simulink model "rbarm_plan_control_backup"  (R2021a)
settings: Solver=VariableStepAuto  StartTime=0.0  StopTime=6  FixedStep=0.00001  RelTol=1e-3
model workspace: external: MATLAB File E:\attachments\attachments\Assem1_DataFile1.m (data not in the file)
undefined symbols (not defined in the file): smiData, X, Y, Z
libraries: sm_lib x20, nesl_utility x8, simulink x1
settings Model: Creator=Admin  LastModifiedBy=Admin

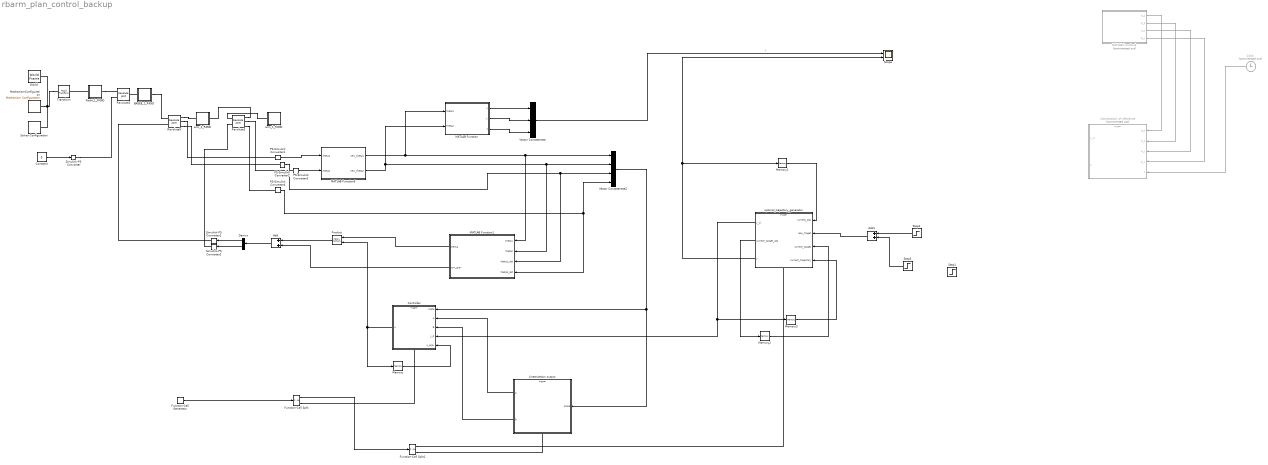
== system rbarm_plan_control_backup ==
  Add : Sum
  Add1 : Sum
  BASEE_1_RIGID : Subsystem
  Clock : Clock  Commented=on
  Constant : Constant  Value=0
  Controller : Subsystem  TreatAsAtomicUnit=on
  Demux : Demux  Outputs=2
  Function-Call Generator : simulink/Ports & Subsystems/Function-Call Generator  sample_time=0.01  numberOfIterations=1  DisallowWideOutput=off
  Function-Call Split : FunctionCallSplit  IconShape=distinctive  NumOutputPorts=2  OutputPortLayout=default
  Function-Call Split1 : FunctionCallSplit  IconShape=distinctive  NumOutputPorts=2  OutputPortLayout=default
  Linearization output : Subsystem  TreatAsAtomicUnit=on
  MATLAB Function : MATLAB Function  TreatAsAtomicUnit=on
  MATLAB Function1 : MATLAB Function  TreatAsAtomicUnit=on
  MATLAB Function3 : MATLAB Function  Commented=on  TreatAsAtomicUnit=on
  MATLAB Function6 : MATLAB Function  TreatAsAtomicUnit=on
  MechanismConfiguration : sm_lib/Utilities/Mechanism Configuration  UniformGravity=Constant  GravityVector=[0 0 9.80665]  GravityVectorUnits=m/s^2  GravityUnits=m/s^2  LinearizationDelta=0.001  JointModeTransitionNonlinearIterations=2
  Memory : Memory  InitialCondition=[0;0]
  Memory1 : Memory  InitialCondition=[0;0;0.24]
  Memory2 : Memory  InitialCondition=[0;0;0.24]
  Memory3 : Memory  InitialCondition=zeros(600,1)
  PS-Simulink Converter{1..4} (4 alike) : nesl_utility/PS-Simulink Converter  PhysicalDomain=network_engine_domain  SubClassName=ps_output  LeftPortType=input  RightPortType=output  PseudoPeriodic=off  Frequencies=[]  Unit=inherit  AffineConversion=off
      settings: SourceProductBaseCode=PW,SS
  Part4_1_RIGID : Subsystem
  Product : Product  Multiplication=Matrix(*)
  Revolute2 : sm_lib/Joints/Revolute Joint  JointMode=Normal  SenseConstraintForce=off  SenseConstraintForceX=off  SenseConstraintForceY=off  SenseConstraintForceZ=off  SenseConstraintTorque=off  SenseConstraintTorqueX=off  SenseConstraintTorqueY=off  SenseConstraintTorqueZ=off  SenseTotalForce=off  SenseTotalForceX=off  SenseTotalForceY=off  SenseTotalForceZ=off  SenseTotalTorque=off  SenseTotalTorqueX=off  SenseTotalTorqueY=off  SenseTotalTorqueZ=off  CompositeWrenchDir=FollowerOnBase  CompositeWrenchFrame=BaseFrame  EquilibriumPosition=0  EquilibriumPositionUnits=deg  SpringStiffness=0  SpringStiffnessUnits=N*m/deg  DampingCoefficient=100  DampingCoefficientUnits=N*m/(deg/s)  TorqueActuationMode=ComputedTorque  MotionActuationMode=InputMotion  SensePosition=off  SenseVelocity=off  SenseAcceleration=off  SenseTorqueForce=off  SenseLowerLimitTorqueForce=off  SenseUpperLimitTorqueForce=off  LowerLimitSpecify=off  LowerLimitBound=-90  LowerLimitBoundUnits=deg  LowerLimitStiffness=1e4  LowerLimitStiffnessUnits=N*m/deg  LowerLimitDamping=10  LowerLimitDampingUnits=N*m/(deg/s)  LowerLimitTransitionRegionWidth=0.1  LowerLimitTransitionRegionWidthUnits=deg  UpperLimitSpecify=off  UpperLimitBound=90  UpperLimitBoundUnits=deg  UpperLimitStiffness=1e4  UpperLimitStiffnessUnits=N*m/deg  UpperLimitDamping=10  UpperLimitDampingUnits=N*m/(deg/s)  UpperLimitTransitionRegionWidth=0.1  UpperLimitTransitionRegionWidthUnits=deg  PositionTargetSpecify=off  PositionTargetPriority=Low  PositionTargetValue=smiData.RevoluteJoint(3).Rz.Pos  PositionTargetValueUnits=deg  VelocityTargetSpecify=off  VelocityTargetPriority=High  VelocityTargetValue=0  VelocityTargetValueUnits=deg/s
  Revolute3 : sm_lib/Joints/Revolute Joint  JointMode=Normal  SenseConstraintForce=off  SenseConstraintForceX=off  SenseConstraintForceY=off  SenseConstraintForceZ=off  SenseConstraintTorque=off  SenseConstraintTorqueX=off  SenseConstraintTorqueY=off  SenseConstraintTorqueZ=off  SenseTotalForce=off  SenseTotalForceX=off  SenseTotalForceY=off  SenseTotalForceZ=off  SenseTotalTorque=off  SenseTotalTorqueX=off  SenseTotalTorqueY=off  SenseTotalTorqueZ=off  CompositeWrenchDir=FollowerOnBase  CompositeWrenchFrame=BaseFrame  EquilibriumPosition=0  EquilibriumPositionUnits=deg  SpringStiffness=0  SpringStiffnessUnits=N*m/deg  DampingCoefficient=0  DampingCoefficientUnits=N*m/(deg/s)  TorqueActuationMode=InputTorque  MotionActuationMode=ComputedMotion  SensePosition=on  SenseVelocity=on  SenseAcceleration=off  SenseTorqueForce=off  SenseLowerLimitTorqueForce=off  SenseUpperLimitTorqueForce=off  LowerLimitSpecify=off  LowerLimitBound=-90  LowerLimitBoundUnits=deg  LowerLimitStiffness=1e4  LowerLimitStiffnessUnits=N*m/deg  LowerLimitDamping=10  LowerLimitDampingUnits=N*m/(deg/s)  LowerLimitTransitionRegionWidth=0.1  LowerLimitTransitionRegionWidthUnits=deg  UpperLimitSpecify=off  UpperLimitBound=90  UpperLimitBoundUnits=deg  UpperLimitStiffness=1e4  UpperLimitStiffnessUnits=N*m/deg  UpperLimitDamping=10  UpperLimitDampingUnits=N*m/(deg/s)  UpperLimitTransitionRegionWidth=0.1  UpperLimitTransitionRegionWidthUnits=deg  PositionTargetSpecify=off  PositionTargetPriority=Low  PositionTargetValue=smiData.RevoluteJoint(4).Rz.Pos  PositionTargetValueUnits=deg  VelocityTargetSpecify=off  VelocityTargetPriority=High  VelocityTargetValue=0  VelocityTargetValueUnits=deg/s
  Revolute5 : sm_lib/Joints/Revolute Joint  JointMode=Normal  SenseConstraintForce=off  SenseConstraintForceX=off  SenseConstraintForceY=off  SenseConstraintForceZ=off  SenseConstraintTorque=off  SenseConstraintTorqueX=off  SenseConstraintTorqueY=off  SenseConstraintTorqueZ=off  SenseTotalForce=off  SenseTotalForceX=off  SenseTotalForceY=off  SenseTotalForceZ=off  SenseTotalTorque=off  SenseTotalTorqueX=off  SenseTotalTorqueY=off  SenseTotalTorqueZ=off  CompositeWrenchDir=FollowerOnBase  CompositeWrenchFrame=BaseFrame  EquilibriumPosition=0  EquilibriumPositionUnits=deg  SpringStiffness=0  SpringStiffnessUnits=N*m/deg  DampingCoefficient=0  DampingCoefficientUnits=N*m/(deg/s)  TorqueActuationMode=InputTorque  MotionActuationMode=ComputedMotion  SensePosition=on  SenseVelocity=on  SenseAcceleration=off  SenseTorqueForce=off  SenseLowerLimitTorqueForce=off  SenseUpperLimitTorqueForce=off  LowerLimitSpecify=off  LowerLimitBound=-90  LowerLimitBoundUnits=deg  LowerLimitStiffness=1e4  LowerLimitStiffnessUnits=N*m/deg  LowerLimitDamping=10  LowerLimitDampingUnits=N*m/(deg/s)  LowerLimitTransitionRegionWidth=0.1  LowerLimitTransitionRegionWidthUnits=deg  UpperLimitSpecify=off  UpperLimitBound=90  UpperLimitBoundUnits=deg  UpperLimitStiffness=1e4  UpperLimitStiffnessUnits=N*m/deg  UpperLimitDamping=10  UpperLimitDampingUnits=N*m/(deg/s)  UpperLimitTransitionRegionWidth=0.1  UpperLimitTransitionRegionWidthUnits=deg  PositionTargetSpecify=off  PositionTargetPriority=Low  PositionTargetValue=smiData.RevoluteJoint(6).Rz.Pos  PositionTargetValueUnits=deg  VelocityTargetSpecify=off  VelocityTargetPriority=High  VelocityTargetValue=0  VelocityTargetValueUnits=deg/s
  Scope : Scope  NumInputPorts=2
  Simulink-PS Converter : nesl_utility/Simulink-PS Converter  PhysicalDomain=network_engine_domain  SubClassName=ps_input  LeftPortType=input  RightPortType=output  PseudoPeriodic=off  Frequencies=[]  NoiseDistribution=none  NoiseParameters=[]  Unit=1  AffineConversion=off  FilteringAndDerivatives=provide  SimscapeFilterOrder=1  InputFilterTimeConstant=0.001  UdotUserProvided=0
      settings: SourceProductBaseCode=PW,SS
  Simulink-PS Converter1 : nesl_utility/Simulink-PS Converter  PhysicalDomain=network_engine_domain  SubClassName=ps_input  LeftPortType=input  RightPortType=output  PseudoPeriodic=off  Frequencies=[]  NoiseDistribution=none  NoiseParameters=[]  Unit=1  AffineConversion=off  FilteringAndDerivatives=provide  SimscapeFilterOrder=1  InputFilterTimeConstant=0.001  UdotUserProvided=0
      settings: SourceProductBaseCode=PW,SS
  Simulink-PS Converter2 : nesl_utility/Simulink-PS Converter  PhysicalDomain=network_engine_domain  SubClassName=ps_input  LeftPortType=input  RightPortType=output  PseudoPeriodic=off  Frequencies=[]  NoiseDistribution=none  NoiseParameters=[]  Unit=1  AffineConversion=off  FilteringAndDerivatives=provide  SimscapeFilterOrder=1  InputFilterTimeConstant=0.001  UdotUserProvided=0
      settings: SourceProductBaseCode=PW,SS
  Solver Configuration : nesl_utility/Solver Configuration  PhysicalDomain=network_engine_domain  SubClassName=solver  LeftPortType=input  RightPortType=generic  Tones=[]  Harmonics=[]  SimulateNoise=off  Profile=off  UseLocalSampling=off  EnableSwitchedLinearOptims=on  FrequencyDomain=off  UseCCode=off  RelTol=0.001  AbsTol=1e-06  MinStep=1e-09  ToWorkspace=off  RevertToSquareIcSolve=off  NumHomotopyIterations=100  PhasorMode=off  PhasorModeNumHarmonics=1  DoDC=off  ResidualTolerance=1e-09  UseLocalSolver=off  LocalSolverChoice=NE_BACKWARD_EULER_ADVANCER  LocalSolverSampleTime=0.001  DoFixedCost=off  MaxNonlinIter=3  MaxModeIter=2  ComputeImpulses=off  ImpulseIterations=2  LinearAlgebra=auto  EquationFormulation=NE_TIME_EF  DelaysMemoryBudget=1024  AutomaticFiltering=on  FilteringTimeConstant=0.001  PartitionStorageMethod=AS_NEEDED  PartitionMemoryBudget=1024  PartitionMethod=ROBUST
      settings: SourceProductBaseCode=PW,SS
  Step1 : Step  Time=3  Before=[0;0;0]  After=[0;0.0439;-0.0557]  SampleTime=0
  Step2 : Step  Time=0.5  Before=[0;0;0.24]  After=[0;-0.1639;0.1]  SampleTime=0
  Step3 : Step  Time=3  Before=[0;0;0]  After=[0;0.0439;-0.2]  SampleTime=0
  Transform : sm_lib/Frames and Transforms/Rigid Transform  TranslationMethod=Cartesian  TranslationStandardOffset=0  TranslationLengthUnit=mm  TranslationStandardAxis=+Z  TranslationCartesianOffset=smiData.RigidTransform(19).translation  TranslationROffset=0  TranslationROffsetUnits=m  TranslationZOffset=0  TranslationZOffsetUnits=m  TranslationThetaOffset=0  TranslationThetaOffsetUnits=deg  RotationMethod=StandardAxis  RotationAngleUnits=rad  RotationStandardAxis=+Z  RotationAngle=smiData.RigidTransform(19).angle  RotationArbitraryAxis=smiData.RigidTransform(19).axis  FollAlignAxisA=+X  BaseAlignAxisA=+Y  FollAlignAxisB=+Y  BaseAlignAxisB=+Z  RotationSequenceAxes=FollowerAxes  RotationSequence=XYX  RotationSequenceAngles=[0 0 0]  RotationSequenceAnglesUnits=deg  RotationMatrix=[1 0 0; 0 1 0; 0 0 1]
  Vector Concatenate : Concatenate  NumInputs=3
  Vector Concatenate2 : Concatenate  NumInputs=4
  World : sm_lib/Frames and Transforms/World Frame
  arm_1_RIGID : Subsystem
  arm_2_RIGID : Subsystem
  discretization of reference : Subsystem  Commented=on  TreatAsAtomicUnit=on
  optimal_trajectory_generator : Subsystem  TreatAsAtomicUnit=on
  wires:
  Constant/1 -> Simulink-PS Converter/1
  MATLAB Function1/2(cori_grav) -> Add/2
  Add/1 -> Demux/1
  Demux/1 -> Simulink-PS Converter1/1
  Demux/2 -> Simulink-PS Converter2/1
  MATLAB Function/2(y) -> Vector Concatenate/2
  MATLAB Function/1(x) -> Vector Concatenate/1
  MATLAB Function/3(z) -> Vector Concatenate/3
  MATLAB Function1/1(inertia) -> Product/1
  MATLAB Function3/1(a_z) -> discretization of reference/1(a_z)
  MATLAB Function3/2(b_z) -> discretization of reference/2(b_z)
  MATLAB Function3/3(a_y) -> discretization of reference/3(a_y)
  MATLAB Function3/4(b_y) -> discretization of reference/4(b_y)
  Clock/1 -> discretization of reference/5(t)
  Product/1 -> Add/1
  PS-Simulink Converter3/1 -> MATLAB Function6/2(theta2)
  PS-Simulink Converter1/1 -> MATLAB Function6/1(theta1)
  MATLAB Function6/1(new_theta1) -> MATLAB Function1/1(theta1), Vector Concatenate2/1, MATLAB Function/1(theta1)
  MATLAB Function6/2(new_theta2) -> MATLAB Function/2(theta2), MATLAB Function1/2(theta2), Vector Concatenate2/2
  Controller/1(u) -> Product/2, Memory/1
  Function-Call Generator/1 -> Function-Call Split/1
  Function-Call Split/2 -> Controller/Trigger
  Linearization output/1(A) -> Controller/2(A)
  Linearization output/2(B) -> Controller/3(B)
  Vector Concatenate2/1 -> Linearization output/1(state), Controller/1(state)
  Function-Call Split/1 -> Function-Call Split1/1
  PS-Simulink Converter2/1 -> MATLAB Function1/3(theta1_dot), Vector Concatenate2/3
  PS-Simulink Converter4/1 -> MATLAB Function1/4(theta2_dot), Vector Concatenate2/4
  Vector Concatenate/1 -> Scope/1  "Y"
  Memory/1 -> Controller/5(u_prev)
  Step2/1 -> Add1/1
  Add1/1 -> optimal_trajectory_generator/2(new_traget)
  optimal_trajectory_generator/2(current_target_pos) -> Memory2/1
  Memory2/1 -> optimal_trajectory_generator/3(current_target)
  Memory3/1 -> optimal_trajectory_generator/4(current_trajectory)
  optimal_trajectory_generator/3(y) -> Scope/2, Memory1/1
  Function-Call Split1/1 -> optimal_trajectory_generator/Trigger
  Function-Call Split1/2 -> Linearization output/Trigger
  optimal_trajectory_generator/1(y_d) -> Controller/4(y_d), Memory3/1
  Memory1/1 -> optimal_trajectory_generator/1(current_pos)
  Step3/1 -> Add1/2
  connections:
  Transform/LConn1 -- MechanismConfiguration/RConn1 -- Solver Configuration/RConn1 -- World/RConn1
  BASEE_1_RIGID/RConn1 -- Revolute5/LConn1
  Revolute5/RConn1 -- arm_2_RIGID/LConn1
  Part4_1_RIGID/LConn1 -- Transform/RConn1
  Part4_1_RIGID/RConn1 -- Revolute2/LConn1
  BASEE_1_RIGID/LConn1 -- Revolute2/RConn1
  Revolute3/LConn1 -- arm_1_RIGID/LConn1
  Revolute3/RConn1 -- arm_2_RIGID/RConn1
  Simulink-PS Converter/RConn1 -- Revolute2/LConn2
  Revolute5/RConn2 -- PS-Simulink Converter1/LConn1
  Revolute5/RConn3 -- PS-Simulink Converter2/LConn1
  Revolute3/RConn2 -- PS-Simulink Converter3/LConn1
  Revolute3/RConn3 -- PS-Simulink Converter4/LConn1
  Simulink-PS Converter1/RConn1 -- Revolute5/LConn2
  Simulink-PS Converter2/RConn1 -- Revolute3/LConn2

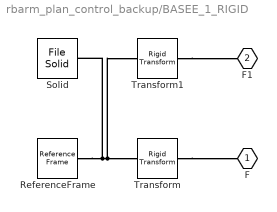
== system rbarm_plan_control_backup/BASEE_1_RIGID ==
  ReferenceFrame : sm_lib/Frames and Transforms/Reference Frame
  Solid : sm_lib/Body Elements/File Solid  ExtGeomFileName=BASEE_Default_sldprt.STEP  UnitType=FromFile  ExtGeomFileUnits=m  StepReaderType=HEX  ExportConvexHullGeometry=off  InertiaType=CalculateFromGeometry  Mass=smiData.Solid(7).mass  MassUnits=kg  CenterOfMass=smiData.Solid(7).CoM  CenterOfMassUnits=mm  MomentsOfInertia=smiData.Solid(7).MoI  MomentsOfInertiaUnits=kg*mm^2  ProductsOfInertia=smiData.Solid(7).PoI  ProductsOfInertiaUnits=kg*mm^2  BasedOnType=Density  Density=8000  DensityUnits=kg/m^3  DoExposeReferenceFrame=on  SerializedFrames=<Frames/>  GraphicType=FromGeometry  MarkerShape=Sphere  MarkerSize=10  GraphicVisPropType=SimpleVisualProperties  GraphicDiffuseColor=smiData.Solid(7).color  GraphicSpecularColor=[0.5 0.5 0.5 1.0]  GraphicAmbientColor=[0.15 0.15 0.15 1.0]  GraphicEmissiveColor=[0.0 0.0 0.0 1.0]  GraphicShininess=75  GraphicOpacity=smiData.Solid(7).opacity
  Transform : sm_lib/Frames and Transforms/Rigid Transform  TranslationMethod=Cartesian  TranslationStandardOffset=0  TranslationLengthUnit=mm  TranslationStandardAxis=+Z  TranslationCartesianOffset=smiData.RigidTransform(6).translation  TranslationROffset=0  TranslationROffsetUnits=m  TranslationZOffset=0  TranslationZOffsetUnits=m  TranslationThetaOffset=0  TranslationThetaOffsetUnits=deg  RotationMethod=ArbitraryAxis  RotationAngleUnits=rad  RotationStandardAxis=+Z  RotationAngle=smiData.RigidTransform(6).angle  RotationArbitraryAxis=smiData.RigidTransform(6).axis  FollAlignAxisA=+X  BaseAlignAxisA=+Y  FollAlignAxisB=+Y  BaseAlignAxisB=+Z  RotationSequenceAxes=FollowerAxes  RotationSequence=XYX  RotationSequenceAngles=[0 0 0]  RotationSequenceAnglesUnits=deg  RotationMatrix=[1 0 0; 0 1 0; 0 0 1]
  Transform1 : sm_lib/Frames and Transforms/Rigid Transform  TranslationMethod=Cartesian  TranslationStandardOffset=0  TranslationLengthUnit=mm  TranslationStandardAxis=+Z  TranslationCartesianOffset=smiData.RigidTransform(15).translation  TranslationROffset=0  TranslationROffsetUnits=m  TranslationZOffset=0  TranslationZOffsetUnits=m  TranslationThetaOffset=0  TranslationThetaOffsetUnits=deg  RotationMethod=ArbitraryAxis  RotationAngleUnits=rad  RotationStandardAxis=+Z  RotationAngle=smiData.RigidTransform(15).angle  RotationArbitraryAxis=smiData.RigidTransform(15).axis  FollAlignAxisA=+X  BaseAlignAxisA=+Y  FollAlignAxisB=+Y  BaseAlignAxisB=+Z  RotationSequenceAxes=FollowerAxes  RotationSequence=XYX  RotationSequenceAngles=[0 0 0]  RotationSequenceAnglesUnits=deg  RotationMatrix=[1 0 0; 0 1 0; 0 0 1]
  F : PMIOPort  Side=Left
  F1 : PMIOPort  Port=2  Side=Right
  connections:
  Solid/RConn1 -- ReferenceFrame/RConn1 -- Transform/LConn1 -- Transform1/LConn1
  Transform/RConn1 -- F/RConn1
  Transform1/RConn1 -- F1/RConn1

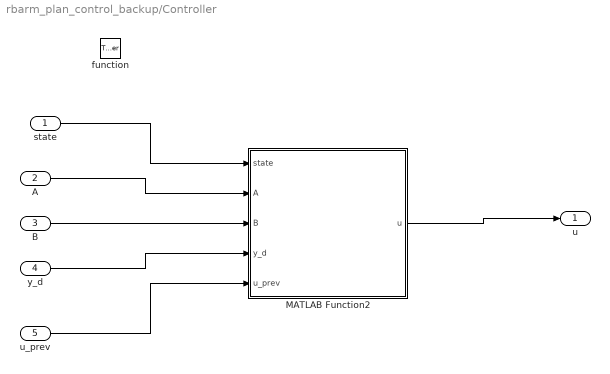
== system rbarm_plan_control_backup/Controller ==
  state : Inport
  A : Inport  Port=2
  B : Inport  Port=3
  y_d : Inport  Port=4
  u_prev : Inport  Port=5
  function : TriggerPort  TriggerType=function-call  VariantControl=(inherit)
  MATLAB Function2 : MATLAB Function  TreatAsAtomicUnit=on
  u : Outport
  wires:
  MATLAB Function2/1(u) -> u/1
  state/1 -> MATLAB Function2/1(state)
  A/1 -> MATLAB Function2/2(A)
  B/1 -> MATLAB Function2/3(B)
  y_d/1 -> MATLAB Function2/4(y_d)
  u_prev/1 -> MATLAB Function2/5(u_prev)

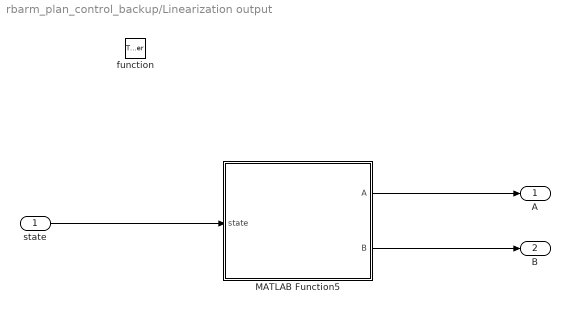
== system rbarm_plan_control_backup/Linearization output ==
  state : Inport
  function : TriggerPort  TriggerType=function-call  VariantControl=(inherit)
  MATLAB Function5 : MATLAB Function  TreatAsAtomicUnit=on
  A : Outport
  B : Outport  Port=2
  wires:
  state/1 -> MATLAB Function5/1(state)
  MATLAB Function5/1(A) -> A/1
  MATLAB Function5/2(B) -> B/1

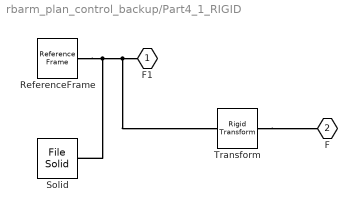
== system rbarm_plan_control_backup/Part4_1_RIGID ==
  ReferenceFrame : sm_lib/Frames and Transforms/Reference Frame
  Solid : sm_lib/Body Elements/File Solid  ExtGeomFileName=Part4_Default_sldprt.STEP  UnitType=FromFile  ExtGeomFileUnits=m  StepReaderType=HEX  ExportConvexHullGeometry=off  InertiaType=CalculateFromGeometry  Mass=smiData.Solid(6).mass  MassUnits=kg  CenterOfMass=smiData.Solid(6).CoM  CenterOfMassUnits=mm  MomentsOfInertia=smiData.Solid(6).MoI  MomentsOfInertiaUnits=kg*mm^2  ProductsOfInertia=smiData.Solid(6).PoI  ProductsOfInertiaUnits=kg*mm^2  BasedOnType=Density  Density=8000  DensityUnits=kg/m^3  DoExposeReferenceFrame=on  SerializedFrames=<Frames/>  GraphicType=FromGeometry  MarkerShape=Sphere  MarkerSize=10  GraphicVisPropType=SimpleVisualProperties  GraphicDiffuseColor=smiData.Solid(6).color  GraphicSpecularColor=[0.5 0.5 0.5 1.0]  GraphicAmbientColor=[0.15 0.15 0.15 1.0]  GraphicEmissiveColor=[0.0 0.0 0.0 1.0]  GraphicShininess=75  GraphicOpacity=smiData.Solid(6).opacity
  Transform : sm_lib/Frames and Transforms/Rigid Transform  TranslationMethod=Cartesian  TranslationStandardOffset=0  TranslationLengthUnit=mm  TranslationStandardAxis=+Z  TranslationCartesianOffset=smiData.RigidTransform(5).translation  TranslationROffset=0  TranslationROffsetUnits=m  TranslationZOffset=0  TranslationZOffsetUnits=m  TranslationThetaOffset=0  TranslationThetaOffsetUnits=deg  RotationMethod=ArbitraryAxis  RotationAngleUnits=rad  RotationStandardAxis=+Z  RotationAngle=smiData.RigidTransform(5).angle  RotationArbitraryAxis=smiData.RigidTransform(5).axis  FollAlignAxisA=+X  BaseAlignAxisA=+Y  FollAlignAxisB=+Y  BaseAlignAxisB=+Z  RotationSequenceAxes=FollowerAxes  RotationSequence=XYX  RotationSequenceAngles=[0 0 0]  RotationSequenceAnglesUnits=deg  RotationMatrix=[1 0 0; 0 1 0; 0 0 1]
  F1 : PMIOPort  Side=Left
  F : PMIOPort  Port=2  Side=Right
  connections:
  Solid/RConn1 -- ReferenceFrame/RConn1 -- Transform/LConn1 -- F1/RConn1
  Transform/RConn1 -- F/RConn1

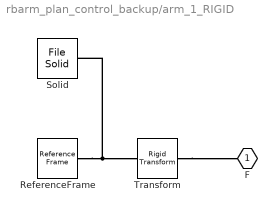
== system rbarm_plan_control_backup/arm_1_RIGID ==
  ReferenceFrame : sm_lib/Frames and Transforms/Reference Frame
  Solid : sm_lib/Body Elements/File Solid  ExtGeomFileName=arm_Default_sldprt.STEP  UnitType=FromFile  ExtGeomFileUnits=m  StepReaderType=HEX  ExportConvexHullGeometry=off  InertiaType=CalculateFromGeometry  Mass=smiData.Solid(3).mass  MassUnits=kg  CenterOfMass=smiData.Solid(3).CoM  CenterOfMassUnits=mm  MomentsOfInertia=smiData.Solid(3).MoI  MomentsOfInertiaUnits=kg*mm^2  ProductsOfInertia=smiData.Solid(3).PoI  ProductsOfInertiaUnits=kg*mm^2  BasedOnType=Density  Density=8000  DensityUnits=kg/m^3  DoExposeReferenceFrame=on  SerializedFrames=<Frames/>  GraphicType=FromGeometry  MarkerShape=Sphere  MarkerSize=10  GraphicVisPropType=SimpleVisualProperties  GraphicDiffuseColor=smiData.Solid(3).color  GraphicSpecularColor=[0.5 0.5 0.5 1.0]  GraphicAmbientColor=[0.15 0.15 0.15 1.0]  GraphicEmissiveColor=[0.0 0.0 0.0 1.0]  GraphicShininess=75  GraphicOpacity=smiData.Solid(3).opacity
  Transform : sm_lib/Frames and Transforms/Rigid Transform  TranslationMethod=Cartesian  TranslationStandardOffset=0  TranslationLengthUnit=mm  TranslationStandardAxis=+Z  TranslationCartesianOffset=smiData.RigidTransform(11).translation  TranslationROffset=0  TranslationROffsetUnits=m  TranslationZOffset=0  TranslationZOffsetUnits=m  TranslationThetaOffset=0  TranslationThetaOffsetUnits=deg  RotationMethod=ArbitraryAxis  RotationAngleUnits=rad  RotationStandardAxis=+Z  RotationAngle=smiData.RigidTransform(11).angle  RotationArbitraryAxis=smiData.RigidTransform(11).axis  FollAlignAxisA=+X  BaseAlignAxisA=+Y  FollAlignAxisB=+Y  BaseAlignAxisB=+Z  RotationSequenceAxes=FollowerAxes  RotationSequence=XYX  RotationSequenceAngles=[0 0 0]  RotationSequenceAnglesUnits=deg  RotationMatrix=[1 0 0; 0 1 0; 0 0 1]
  F : PMIOPort  Side=Left
  connections:
  Solid/RConn1 -- ReferenceFrame/RConn1 -- Transform/LConn1
  Transform/RConn1 -- F/RConn1

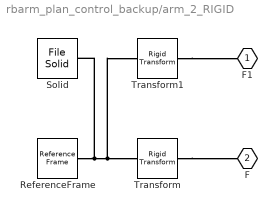
== system rbarm_plan_control_backup/arm_2_RIGID ==
  ReferenceFrame : sm_lib/Frames and Transforms/Reference Frame
  Solid : sm_lib/Body Elements/File Solid  ExtGeomFileName=arm_Default_sldprt.STEP  UnitType=FromFile  ExtGeomFileUnits=m  StepReaderType=HEX  ExportConvexHullGeometry=off  InertiaType=CalculateFromGeometry  Mass=smiData.Solid(3).mass  MassUnits=kg  CenterOfMass=smiData.Solid(3).CoM  CenterOfMassUnits=mm  MomentsOfInertia=smiData.Solid(3).MoI  MomentsOfInertiaUnits=kg*mm^2  ProductsOfInertia=smiData.Solid(3).PoI  ProductsOfInertiaUnits=kg*mm^2  BasedOnType=Density  Density=8000  DensityUnits=kg/m^3  DoExposeReferenceFrame=on  SerializedFrames=<Frames><Frame><Id>Frame1</Id><Value><Name>F1</Name><Origin><Source>CenterOfMassFrame</Source><FeatureName></FeatureName></Origin><PrimaryAxis><DefinedDirection>+Z</DefinedDirection><Source>CenterOfMassFrame</Source><SourceDirection>+Z</SourceDirection><FeatureName></FeatureName></PrimaryAxis><SecondaryAxis><DefinedDirection>+X</DefinedDirection><Source>ReferenceFrame</Source><SourceDirection>+X</SourceDirection><FeatureName></FeatureName></SecondaryAxis></Value></Frame></Frames>  GraphicType=FromGeometry  MarkerShape=Sphere  MarkerSize=10  GraphicVisPropType=SimpleVisualProperties  GraphicDiffuseColor=smiData.Solid(3).color  GraphicSpecularColor=[0.5 0.5 0.5 1.0]  GraphicAmbientColor=[0.15 0.15 0.15 1.0]  GraphicEmissiveColor=[0.0 0.0 0.0 1.0]  GraphicShininess=75  GraphicOpacity=smiData.Solid(3).opacity
  Transform : sm_lib/Frames and Transforms/Rigid Transform  TranslationMethod=Cartesian  TranslationStandardOffset=0  TranslationLengthUnit=mm  TranslationStandardAxis=+Z  TranslationCartesianOffset=smiData.RigidTransform(12).translation  TranslationROffset=0  TranslationROffsetUnits=m  TranslationZOffset=0  TranslationZOffsetUnits=m  TranslationThetaOffset=0  TranslationThetaOffsetUnits=deg  RotationMethod=ArbitraryAxis  RotationAngleUnits=rad  RotationStandardAxis=+Z  RotationAngle=smiData.RigidTransform(12).angle  RotationArbitraryAxis=smiData.RigidTransform(12).axis  FollAlignAxisA=+X  BaseAlignAxisA=+Y  FollAlignAxisB=+Y  BaseAlignAxisB=+Z  RotationSequenceAxes=FollowerAxes  RotationSequence=XYX  RotationSequenceAngles=[0 0 0]  RotationSequenceAnglesUnits=deg  RotationMatrix=[1 0 0; 0 1 0; 0 0 1]
  Transform1 : sm_lib/Frames and Transforms/Rigid Transform  TranslationMethod=Cartesian  TranslationStandardOffset=0  TranslationLengthUnit=mm  TranslationStandardAxis=+Z  TranslationCartesianOffset=smiData.RigidTransform(16).translation  TranslationROffset=0  TranslationROffsetUnits=m  TranslationZOffset=0  TranslationZOffsetUnits=m  TranslationThetaOffset=0  TranslationThetaOffsetUnits=deg  RotationMethod=ArbitraryAxis  RotationAngleUnits=rad  RotationStandardAxis=+Z  RotationAngle=smiData.RigidTransform(16).angle  RotationArbitraryAxis=smiData.RigidTransform(16).axis  FollAlignAxisA=+X  BaseAlignAxisA=+Y  FollAlignAxisB=+Y  BaseAlignAxisB=+Z  RotationSequenceAxes=FollowerAxes  RotationSequence=XYX  RotationSequenceAngles=[0 0 0]  RotationSequenceAnglesUnits=deg  RotationMatrix=[1 0 0; 0 1 0; 0 0 1]
  F1 : PMIOPort  Side=Left
  F : PMIOPort  Port=2  Side=Right
  connections:
  Solid/RConn1 -- Transform/LConn1 -- Transform1/LConn1 -- ReferenceFrame/RConn1
  Transform/RConn1 -- F/RConn1
  Transform1/RConn1 -- F1/RConn1

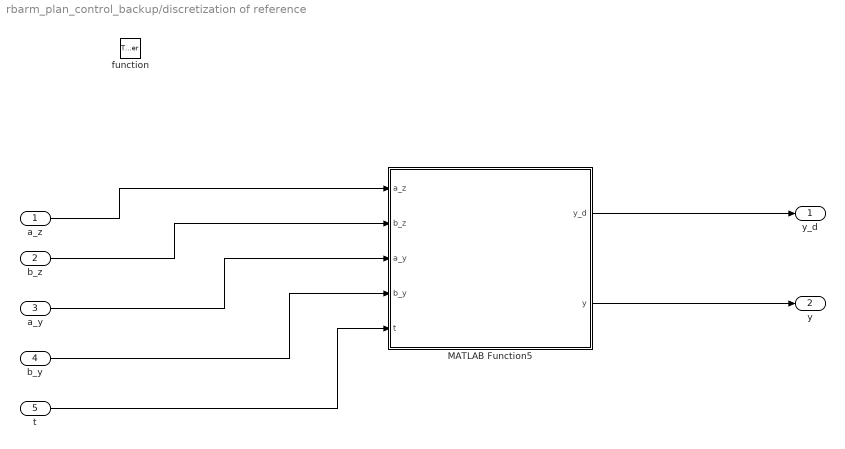
== system rbarm_plan_control_backup/discretization of reference ==
  a_z : Inport
  b_z : Inport  Port=2
  a_y : Inport  Port=3
  b_y : Inport  Port=4
  t : Inport  Port=5
  function : TriggerPort  TriggerType=function-call  VariantControl=(inherit)
  MATLAB Function5 : MATLAB Function  TreatAsAtomicUnit=on
  y_d : Outport
  y : Outport  Port=2
  wires:
  a_z/1 -> MATLAB Function5/1(a_z)
  b_z/1 -> MATLAB Function5/2(b_z)
  a_y/1 -> MATLAB Function5/3(a_y)
  b_y/1 -> MATLAB Function5/4(b_y)
  MATLAB Function5/1(y_d) -> y_d/1
  t/1 -> MATLAB Function5/5(t)
  MATLAB Function5/2(y) -> y/1

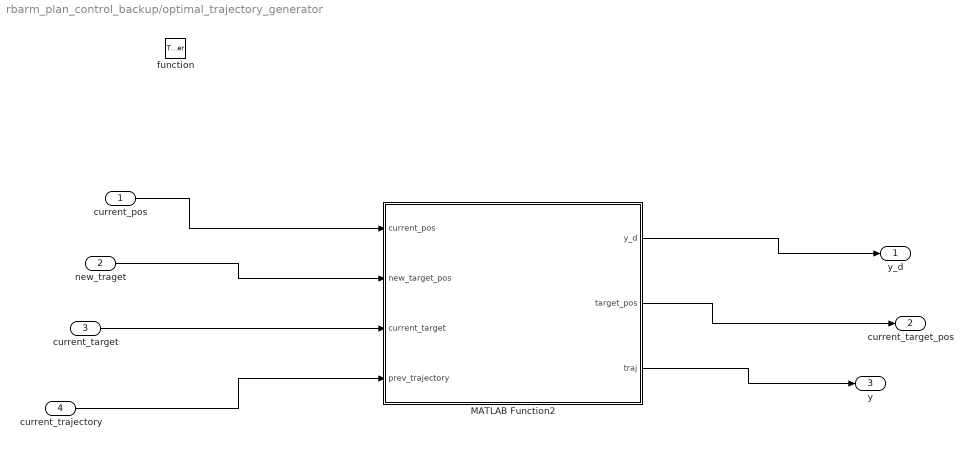
== system rbarm_plan_control_backup/optimal_trajectory_generator ==
  current_pos : Inport
  new_traget : Inport  Port=2
  current_target : Inport  Port=3
  current_trajectory : Inport  Port=4
  function : TriggerPort  TriggerType=function-call  VariantControl=(inherit)
  MATLAB Function2 : MATLAB Function  TreatAsAtomicUnit=on
  y_d : Outport
  current_target_pos : Outport  Port=2
  y : Outport  Port=3
  wires:
  MATLAB Function2/1(y_d) -> y_d/1
  MATLAB Function2/2(target_pos) -> current_target_pos/1
  current_pos/1 -> MATLAB Function2/1(current_pos)
  new_traget/1 -> MATLAB Function2/2(new_target_pos)
  current_target/1 -> MATLAB Function2/3(current_target)
  current_trajectory/1 -> MATLAB Function2/4(prev_trajectory)
  MATLAB Function2/3(traj) -> y/1

== matlab function rbarm_plan_control_backup/Controller/MATLAB Function2 ==
  data: u output; state input; A input; B input; y_d input; u_prev input
function u   = controller(state,A,B,y_d,u_prev)

% Our system after partitioned control
%  d[theta        =  [0  I  [theta      + [0 *u              
%    theta_dot]/dt    0  0]  theta_dot]    I]

% Discretization of the system
A_sys = [zeros(2,2) eye(2);
         zeros(2,4)];
dis_A_sys = expm(A_sys*0.01);

% Approximation of dis_B_sys = integral(expm(A_sys*t),0,0.05,'ArrayValued',true)*[zeros(2,2);eye(2)];

dis_B_sys = (eye(4)*0.01 + A_sys*0.01^2/2 + A_sys^2*0.01^3/6 + A_sys^3*0.01^4/24)*[zeros(2,2);eye(2)]; 

% Cost matrices

R = 0.0001*eye(400);

Q = 50000*eye(600);

% MPC controller design

O = [];
M = [];
L = [];
W1 = [];
T = [];
for i = 1:200
    O = [O;A*dis_A_sys^i];
    temp = zeros(3,400);
    temp2 = zeros(2,400);
    for k = 1:i
        temp(:,2*(k-1)+1:2*k) = A*dis_A_sys^(i-k)*dis_B_sys;
    end 
    
    temp2(:,2*(i-1)+1:2*i) = eye(2);
    if i  > 1
       temp2(:,2*(i-2)+1:2*(i-1)) = -eye(2);
    end
    W1 = [W1;temp2]; 
    M = [M;temp];
    L = [L;B];
    if i == 1
        T = [T; [R(1,1),0; 0, R(2,2)]*u_prev];
    else
        T = [T; zeros(2,1)];
    end
end

s = y_d - O*state - L; 

U = inv(transpose(M)*Q*M + transpose(W1)*R*W1)*(transpose(M)*Q*s+T);

u = U(1:2);

== matlab function rbarm_plan_control_backup/MATLAB Function1 ==
  data: theta1 input; inertia output; theta2 input; theta1_dot input; theta2_dot input; cori_grav output
function [inertia, cori_grav] = partitioned_control(theta1, theta2, theta1_dot, theta2_dot)
inertia = [0.053+0.0352*cos(theta2) ,0.0088+0.0176*cos(theta2);
           0.0176*cos(theta2)+0.0088 ,0.0088];
cori_grav = [2.88*cos(theta1)+1.44*cos(theta1+theta2)+0.016*theta1_dot+0.008*theta2_dot+0.0176*sin(theta2)*theta1_dot^2-0.0176*sin(theta2)*(theta1_dot+theta2_dot)^2+1.44*cos(theta1);
             1.44*cos(theta1+theta2)+0.008*theta1_dot+0.008*theta2_dot+0.0176*sin(theta2)*theta1_dot^2];
inertia = inertia;

== matlab function rbarm_plan_control_backup/MATLAB Function ==
  data: x output; theta1 input; y output; theta2 input; z output
function [x,y,z] = forward_kinematic(theta1, theta2)
x = 0;
y = 0.12*cos(theta1 + theta2) + 0.12*cos(theta1);
z = 0.12*sin(theta1 + theta2) + 0.12*sin(theta1);

== matlab function rbarm_plan_control_backup/Linearization output/MATLAB Function5 ==
  data: state input; A output; B output
function [A,B]  = Linearization(state)

%x = 0;
%y = 0.12*cos(theta1 + theta2) + 0.12*cos(theta1);
%z = 0.12*sin(theta1 + theta2) + 0.12*sin(theta1);

A = [0,0,0,0;
    -0.12*sin(state(1)+state(2))-0.12*sin(state(1)),-0.12*sin(state(1)+state(2)),0,0;
    0.12*cos(state(1)+state(2))+0.12*cos(state(1)), 0.12*cos(state(1)+state(2)),0,0];
temp = [0;
        0.12*cos(state(1)+state(2))+0.12*cos(state(1));
        0.12*sin(state(1)+state(2))+0.12*sin(state(1))];
B = temp - A*state;

== matlab function rbarm_plan_control_backup/MATLAB Function3 ==
  data: a_z output; b_z output; a_y output; b_y output
function [a_z,b_z,a_y,b_y]  = trajectory_generator()
a_z = -0.07;
b_z = 0.24;
a_y = 0.025;
b_y = 0;

== matlab function rbarm_plan_control_backup/optimal_trajectory_generator/MATLAB Function2 ==
  data: current_pos input; y_d output; new_target_pos input; target_pos output; current_target input; prev_trajectory input; traj output
function [y_d,target_pos,traj]  = optimal_trajectory_generator(current_pos,new_target_pos, current_target,prev_trajectory)
% Our system
%    [theta1       =  [theta1      + T*u
%     theta2](k+1)     theta2](k)       
% Output
%     y(k) =  [0
%              0.12*cos(theta1(k) + theta2(k)) + 0.12*cos(theta1(k))
%              0.12*sin(theta1(k) + theta2(k)) + 0.12*sin(theta1(k))]

%  dy(k) =  [0 , 0 , 0
%           -0.12*sin(theta1(k)+theta2(k))-0.12*sin(theta1(k)), -0.12*sin(theta1(k)), 0    *dx(k)
%            0.12*cos(theta1(k)+theta2(k))+0.12*cos(theta1(k)),  0.12*cos(theta1(k)), 0 ]

% 200 step for control horizon (N = 200)


threshold = 0.001;
y_d = zeros(600,1);

if transpose(current_target-new_target_pos)*(current_target-new_target_pos) > threshold
    
    target_pos = new_target_pos;
    
    y1 = current_pos(2);
    z1 = current_pos(3);
    y2 = new_target_pos(2);
    z2 = new_target_pos(3);

    % Angle corresponded to the initial position
    theta2_0 = acos((y1^2+z1^2-2*0.12^2)/(2*0.12^2));
    theta1_0 = acos(y1/((0.12*cos(theta2_0)+0.12)^2+(0.12*sin(theta2_0))^2)^0.5) - acos((0.12*cos(theta2_0)+0.12)/((0.12*cos(theta2_0)+0.12)^2+(0.12*sin(theta2_0))^2)^0.5);
    if (0.12*sin(theta1_0 + theta2_0) + 0.12*sin(theta1_0))*z1 <= 0
        theta2_0 = -theta2_0;
        theta1_0 = -theta1_0;
    end

    % Angle corresponded to the final position
    theta2_N = acos((y2^2+z2^2-2*0.12^2)/(2*0.12^2));
    theta1_N = acos(y2/((0.12*cos(theta2_N)+0.12)^2+(0.12*sin(theta2_N))^2)^0.5) - acos((0.12*cos(theta2_N)+0.12)/((0.12*cos(theta2_N)+0.12)^2+(0.12*sin(theta2_N))^2)^0.5);
    if (0.12*sin(theta1_N + theta2_N) + 0.12*sin(theta1_N))*z2 <= 0
        theta2_N = -theta2_N;
        theta1_N = -theta1_N;
    end

    current_traj = [];
    Jacobian = [];
    current_input = [];

    % Initialize an initial trajectory

    for k = 0:200
            theta = [theta1_0 + (theta1_N-theta1_0)*k/200 ;
                    theta2_0 + (theta2_N-theta2_0)*k/200];
            u = 100*[(theta1_N-theta1_0)/200;
                    (theta2_N-theta2_0)/200];
            y =   [0.12*cos(theta(1) + theta(2)) + 0.12*cos(theta(1));
                  0.12*sin(theta(1) + theta(2)) + 0.12*sin(theta(1))];

            temp  =  [-0.12*sin(theta(1)+theta(2))-0.12*sin(theta(1)), -0.12*sin(theta(1)+theta(2));  
                      0.12*cos(theta(1)+theta(2))+0.12*cos(theta(1)),  0.12*cos(theta(1)+theta(2))]; 
            current_traj = [current_traj;y];
            Jacobian = [Jacobian;temp];
            if k <200
                current_input = [current_input;u];
            end
    end



    dis_A_sys = eye(2);
    dis_B_sys = 0.01*eye(2);
    C = eye(2);

    % Cost matrx
    Q = 100*eye(400);
    R = 0.3*eye(400);
    R2 = 5*eye(2);

    for j = 1:50                     % 50 iterations of ILQR


        % Initialize the matrices
        M = [];
        W1 = [];
        W2 = [];
        T = [];
        N = [];

        for i = 1:200
            temp = zeros(2,400);  
            temp2 = zeros(2,400);
            temp3 = zeros(2,400);
            for k = 1:i
                temp(:,2*(k-1)+1:2*k) = Jacobian(2*i+1:2*(i+1),:)*dis_A_sys^(i-k)*dis_B_sys;
    %               temp(:,2*(k-1)+1:2*k) = C*dis_A_sys^(i-k)*dis_B_sys;
            end 

            temp2(:,2*(i-1)+1:2*i) = eye(2);
            temp3(:,2*(i-1)+1:2*i) = eye(2);
            if i  > 1
               temp2(:,2*(i-2)+1:2*(i-1)) = -eye(2);
               temp3(:,2*(i-2)+1:2*(i-1)) = -eye(2);
            end
            if i == 200
                N = [N;R2];
            else
                N = [N;zeros(2,2)];
            end
            W1 = [W1;temp2]; 
            W2 = [W2;temp3];
            M = [M;temp];

            if i == 1
                T = [T;transpose(Jacobian(3:4,:)*dis_B_sys)*[Q(1,1),0; 0, Q(2,2)]*current_traj(1:2)];
    %               T = [T;transpose(C*dis_B_sys)*[Q(1,1),0; 0, Q(2,2)]*current_traj(1:2)];
            else
                T = [T; zeros(2,1)];
            end

        end

        Q_prime = transpose(W1)*Q*W1;
        R_prime = transpose(W2)*R*W2;
        % Calculating optimal control law

    %     temp1 = pinv(transpose(M)*Q_prime)*transpose(M(598:end,:));
    %     temp2 = pinv(transpose(M)*Q_prime)*T;
    %     lambda = [0;-inv(temp1(599:end,2:end))*(current_traj(602:end)-temp2(599:600))];
    %     delta_u = -transpose(M)*Q_prime*M\(transpose(M)*Q_prime*current_traj(4:end)- T + transpose(M(4:end,:))*lambda); 

    %     temp1 = -inv(N*inv(transpose(M)*Q_prime)*transpose(M(399:end,:)))*N*inv(transpose(M)*Q_prime)*R_prime;
    %     temp2 = -inv(N*inv(transpose(M)*Q_prime)*transpose(M(399:end,:)))*N*(current_traj(3:end)-inv(transpose(M)*Q)*(T-R_prime*current_input));
    %     
    %     delta_u = -inv(transpose(M)*Q_prime*M + R_prime + transpose(M(399:end,:))*temp1)*(transpose(M)*Q_prime*current_traj(3:end)- T + R_prime*current_input +transpose(M(399:end,:))*temp2); 
        K = zeros(400,398);
        K = [K,N];

        a = [transpose(M)*Q_prime*M+R_prime+K,transpose(M(399:end,:));
         M(399:end,:),zeros(2,2)];
        b = -(transpose(M)*Q_prime*current_traj(3:end) - T +R_prime*current_input+N*current_input(399:end)) ;
        b = [b;0;0]; 
        sol = inv(a)*b;
        delta_u = sol(1:400);

        % Recalculate the trajectory
        current_input = current_input +delta_u;
        x = [theta1_0;theta2_0];
        for k = 1:200
            x = dis_A_sys*x + dis_B_sys*current_input(2*k-1:2*k);
            temp =   [0.12*cos(x(1) + x(2)) + 0.12*cos(x(1));
                    0.12*sin(x(1) + x(2)) + 0.12*sin(x(1))];
            temp2 = [-0.12*sin(x(1)+x(2))-0.12*sin(x(1)), -0.12*sin(x(1)+x(2));  
                      0.12*cos(x(1)+x(2))+0.12*cos(x(1)),  0.12*cos(x(1)+x(2))];
            current_traj(2*k+1:2*k+2) = temp;
            Jacobian(2*k+1:2*k+2,:) = temp2;
        end
    %     current_traj(3:end) = current_traj(3:end) + M*delta_u; 
    end

%     y = [];
%     z = [];
%     for i = 1:200
%        y = [y;current_traj(2*i-1)];
%        z = [z;current_traj(2*i)];
%     end
% 
%     plot(y,z)
    for i = 1:200
        y_d(3*(i-1)+1) = 0;
        y_d(3*(i-1)+2:3*i) = current_traj(2*i+1:2*i+2);
    end
    
else
    target_pos = current_target;
    
    if prev_trajectory == zeros(600,1)
        for i = 1:200
            prev_trajectory(3*i-2:3*i) = current_pos;
        end   
    end
    
    y_d(1:597) = prev_trajectory(4:600);
    y_d(598:600) = prev_trajectory(598:600);
    
end

traj = y_d(1:3);

== matlab function rbarm_plan_control_backup/discretization of reference/MATLAB Function5 ==
  data: a_z input; y_d output; b_z input; a_y input; b_y input; t input; y output
function [y_d,y]  = Discretize_desire_output(a_z,b_z,a_y,b_y,t)

%y = a_z*t +b_z

y_d = zeros(600,1);
for j = 1:1:200
    if t+(j/100) < 2
        temp = [0;
               a_y*(t+(j/100))+b_y;
               a_z*(t+(j/100))+b_z];
    elseif t+(j/100) < 3
        temp = [0;
               -1.5*a_y*(t+(j/100)-2)+a_y*2+b_y;
               -1.5*a_z*(t+(j/100)-2)+a_z*2+b_z];
    else
        temp = [0;
               -1.5*a_y+a_y*2+b_y;
               -1.5*a_z+a_z*2+b_z];
    end
    y_d(3*(j-1)+1:3*j) = temp;
end
y = y_d(1:3);

== matlab function rbarm_plan_control_backup/MATLAB Function6 ==
  data: new_theta1 output; theta1 input; new_theta2 output; theta2 input
function [new_theta1, new_theta2] = angle_transform(theta1, theta2)
new_theta1 = theta1 + pi/2;
new_theta2 = theta2;
